simulink model "v07_mux"  (R2019b)
settings: Solver=FixedStepAuto  StartTime=0.0  StopTime=inf  FixedStep=1  MaxStep=1  RelTol=1e-3
settings Model: Creator=MARAT  LastModifiedBy=Marat
settings SFSimCC: CustomCodeUndefinedFunction=UseInterfaceOnly

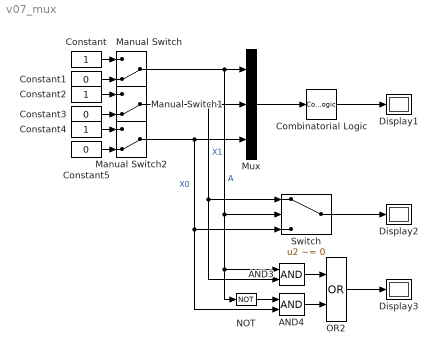
== system v07_mux ==
  AND3 : Logic  IconShape=distinctive  AllPortsSameDT=off  OutDataTypeStr=boolean
  AND4 : Logic  IconShape=distinctive  AllPortsSameDT=off  OutDataTypeStr=boolean
  Combinatorial Logic : CombinatorialLogic  TruthTable=[0; 1; 0; 1; 0; 0; 1; 1]
  Constant : Constant  OutDataTypeStr=boolean
  Constant1 : Constant  Value=0  OutDataTypeStr=boolean
  Constant2 : Constant  OutDataTypeStr=boolean
  Constant3 : Constant  Value=0  OutDataTypeStr=boolean
  Constant4 : Constant  OutDataTypeStr=boolean
  Constant5 : Constant  Value=0  OutDataTypeStr=boolean
  Display1 : Display
  Display2 : Display
  Display3 : Display
  Manual Switch : ManualSwitch  CurrentSetting=0
  Manual Switch1 : ManualSwitch  CurrentSetting=0
  Manual Switch2 : ManualSwitch  CurrentSetting=0
  Mux : Mux  Inputs=3
  NOT : Logic  Operator=NOT  IconShape=distinctive  AllPortsSameDT=off  OutDataTypeStr=boolean
  OR2 : Logic  Operator=OR  IconShape=distinctive  AllPortsSameDT=off  OutDataTypeStr=boolean
  Switch : Switch  Criteria=u2 ~= 0
  wires:
  Mux/1 -> Combinatorial Logic/1
  Combinatorial Logic/1 -> Display1/1
  Constant/1 -> Manual Switch/1
  Constant1/1 -> Manual Switch/2
  Constant3/1 -> Manual Switch1/2
  Constant2/1 -> Manual Switch1/1
  Constant5/1 -> Manual Switch2/2
  Constant4/1 -> Manual Switch2/1
  Manual Switch/1 -> Switch/2, AND3/1, NOT/1, Mux/1  "A"
  Manual Switch1/1 -> AND3/2, Switch/1, Mux/2  "X1"
  Manual Switch2/1 -> Switch/3, AND4/2, Mux/3  "X0"
  NOT/1 -> AND4/1
  Switch/1 -> Display2/1
  OR2/1 -> Display3/1
  AND3/1 -> OR2/1
  AND4/1 -> OR2/2
